simulink model "General_3_2025a"  (R2025a)
settings: Solver=ode45  StartTime=0.0  StopTime=inf  FixedStep=.1  RelTol=1e-3
undefined symbols (not defined in the file or in its folder): CR, DiscIntNeverNeededParam, LF
libraries: instrumentseriallib x3, simulink x2
settings Model: PacingRate=1000  Creator=aceve  LastModifiedBy=diego

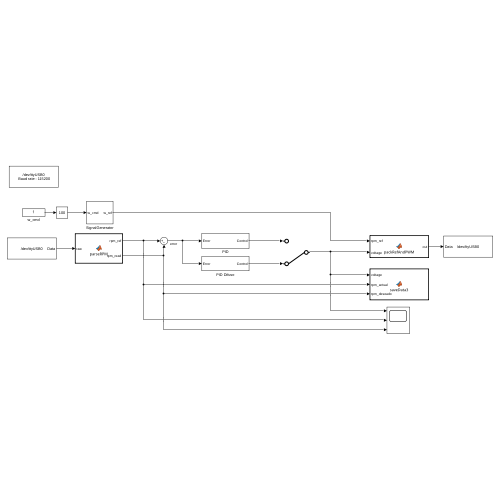
[thumbnail: Simulink's stored preview of the top-level diagram]
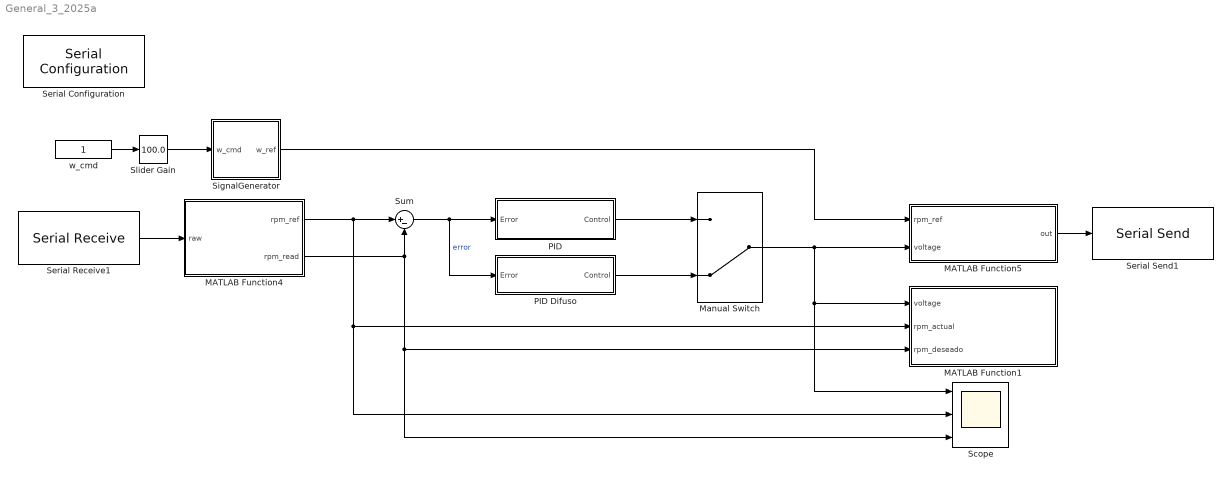
== system General_3_2025a ==
  MATLAB Function1 : MATLAB Function  TreatAsAtomicUnit=on
  MATLAB Function4 : MATLAB Function  TreatAsAtomicUnit=on
  MATLAB Function5 : MATLAB Function  TreatAsAtomicUnit=on
  Manual Switch : ManualSwitch  CurrentSetting=0
  PID : Subsystem
  PID Difuso : Subsystem
  Scope : Scope  NumInputPorts=3
      settings: ActiveDisplayYMinimum=-1  ActiveDisplayYMaximum=1
  Serial Configuration : instrumentseriallib/Serial Configuration  Priority=-200000  PortSel=/dev/ttyUSB0  Port=/dev/ttyUSB0  ComPort=/dev/ttyUSB0  BaudRate=115200  DataBits=8  Parity=none  StopBits=1  ByteOrder=little-endian  FlowControl=none  Timeout=10  SimulateUsing=Interpreted execution  BlockInModel=on  aMode=1
  Serial Receive1 : instrumentseriallib/Serial Receive  Priority=1  PortSel=/dev/ttyUSB0  Port=/dev/ttyUSB0  ComPort=/dev/ttyUSB0  DataType=int16  SaveDataType=uint8  ToggleHeader=off  Header=[]  ToggleDataSize=on  DataSize=[2 1]  ToggleTerminator=off  Terminator=CR/LF ('\r\n')  CustomTerminator=[]  InputFormat=Column major  EnableBlockingMode=on  ActionDataUnavailable=Output last received value  ActionWhenDataUnavailable=Output last received value  CustomValue=0  SampleTime=0.01  SimulateUsing=Interpreted execution  BlockInModel=on  aMode=1  LibraryInUse=instrumentlib
  Serial Send1 : instrumentseriallib/Serial Send  Priority=1  PortSel=/dev/ttyUSB0  Port=/dev/ttyUSB0  ComPort=/dev/ttyUSB0  Header=[]  Terminator=<none>  CustomTerminator=[]  EnableBlockingMode=off  SimulateUsing=Interpreted execution  BlockInModel=on  aMode=1
  SignalGenerator : Subsystem
  Slider Gain : simulink/Math Operations/Slider Gain  gain=100.0  low=100  high=1100
  Sum : Sum  Inputs=|+-
  w_cmd : Constant  SampleTime=-1
  wires:
  PID/1(Control) -> Manual Switch/1
  Sum/1 -> PID Difuso/1(Error), PID/1(Error)  "error"
  w_cmd/1 -> Slider Gain/1
  PID Difuso/1(Control) -> Manual Switch/2
  Serial Receive1/1 -> MATLAB Function4/1(raw)
  MATLAB Function5/1(out) -> Serial Send1/1
  MATLAB Function4/1(rpm_ref) -> Scope/2, MATLAB Function1/2(rpm_actual), Sum/1
  MATLAB Function4/2(rpm_read) -> Sum/2, Scope/3, MATLAB Function1/3(rpm_deseado)
  Manual Switch/1 -> Scope/1, MATLAB Function1/1(voltage), MATLAB Function5/2(voltage)
  Slider Gain/1 -> SignalGenerator/1(w_cmd)
  SignalGenerator/1(w_ref) -> MATLAB Function5/1(rpm_ref)

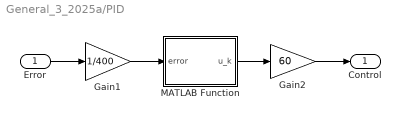
== system General_3_2025a/PID ==
  Error : Inport
  Gain1 : Gain  Gain=1/400
  Gain2 : Gain  Gain=60
  MATLAB Function : MATLAB Function  TreatAsAtomicUnit=on
  Control : Outport
  wires:
  Gain1/1 -> MATLAB Function/1(error)
  MATLAB Function/1(u_k) -> Gain2/1
  Error/1 -> Gain1/1
  Gain2/1 -> Control/1

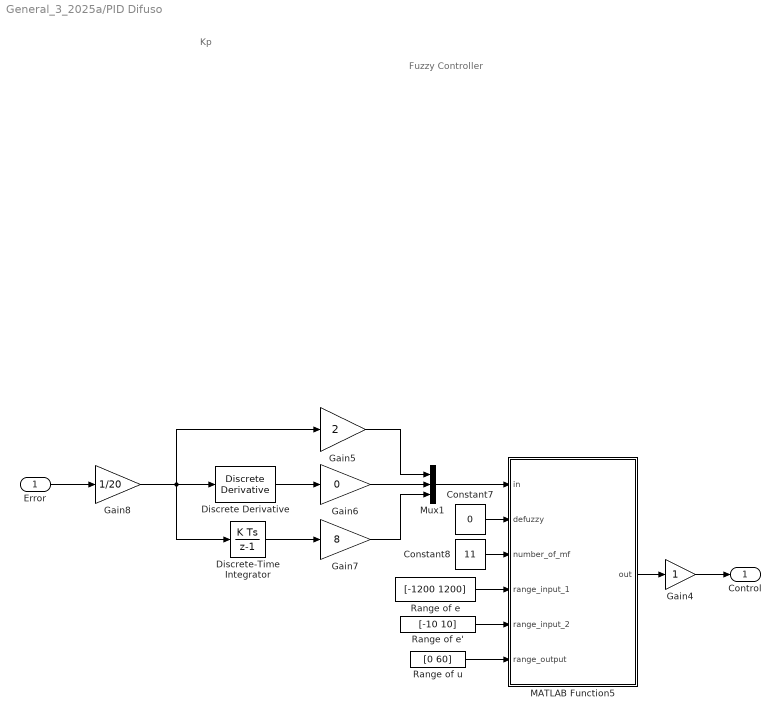
== system General_3_2025a/PID Difuso ==
  note: Fuzzy Controller
  note: Kp
  Error : Inport
  Constant7 : Constant  Value=0
  Constant8 : Constant  Value=11
  Discrete Derivative : simulink/Discrete/Discrete Derivative  gainval=1.0  ICPrevScaledInput=0.0  OutMin=[]  OutMax=[]  OutDataType=fixdt(1, 16)  OutScaling=2^-10  DoSatur=off
  Discrete-Time Integrator : DiscreteIntegrator  SampleTime=0.01  ICPrevOutput=DiscIntNeverNeededParam  ICPrevScaledInput=DiscIntNeverNeededParam
  Gain4 : Gain
  Gain5 : Gain  Gain=2
  Gain6 : Gain  Gain=0
  Gain7 : Gain  Gain=8
  Gain8 : Gain  Gain=1/20
  MATLAB Function5 : MATLAB Function  TreatAsAtomicUnit=on
  Mux1 : Mux  Inputs=3
  Range of e : Constant  Value=[-1200 1200]
  Range of e' : Constant  Value=[-10 10]
  Range of u : Constant  Value=[0 60]
  Control : Outport
  wires:
  Gain7/1 -> Mux1/3
  Range of e/1 -> MATLAB Function5/4(range_input_1)
  Gain8/1 -> Gain5/1, Discrete-Time Integrator/1, Discrete Derivative/1
  Gain6/1 -> Mux1/2
  MATLAB Function5/1(out) -> Gain4/1
  Constant8/1 -> MATLAB Function5/3(number_of_mf)
  Mux1/1 -> MATLAB Function5/1(in)
  Discrete Derivative/1 -> Gain6/1
  Discrete-Time Integrator/1 -> Gain7/1
  Range of e'/1 -> MATLAB Function5/5(range_input_2)
  Range of u/1 -> MATLAB Function5/6(range_output)
  Constant7/1 -> MATLAB Function5/2(defuzzy)
  Gain5/1 -> Mux1/1
  Gain4/1 -> Control/1
  Error/1 -> Gain8/1

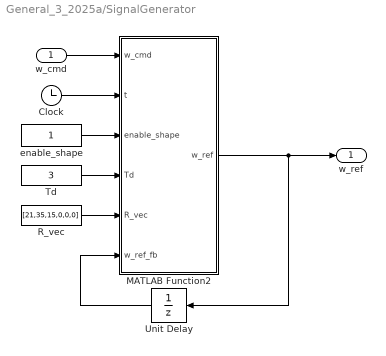
== system General_3_2025a/SignalGenerator ==
  w_cmd : Inport
  Clock : Clock
  MATLAB Function2 : MATLAB Function  TreatAsAtomicUnit=on
  R_vec : Constant  Value=[21,35,15,0,0,0]  SampleTime=-1
  Td : Constant  Value=3  SampleTime=-1
  Unit Delay : UnitDelay  SampleTime=-1  HasFrameUpgradeWarning=on
  enable_shape : Constant  SampleTime=-1
  w_ref : Outport
  wires:
  Clock/1 -> MATLAB Function2/2(t)
  Td/1 -> MATLAB Function2/4(Td)
  enable_shape/1 -> MATLAB Function2/3(enable_shape)
  Unit Delay/1 -> MATLAB Function2/6(w_ref_fb)
  R_vec/1 -> MATLAB Function2/5(R_vec)
  MATLAB Function2/1(w_ref) -> Unit Delay/1, w_ref/1
  w_cmd/1 -> MATLAB Function2/1(w_cmd)

== matlab function General_3_2025a/SignalGenerator/MATLAB Function2 ==
  settings: updateMethod=DISCRETE
  data: w_cmd input; t input; w_ref output; enable_shape input; Td input; R_vec input; w_ref_fb input
function w_ref = BezierRef(w_cmd, t, enable_shape, Td, R_vec, w_ref_fb)
% =================================================================
% VERSIÓN 5 (Coeficientes R_vec y bug de comparación corregidos)
% =================================================================
%
% Entradas:
%   w_cmd     : setpoint deseado (de la GUI)
%   t         : tiempo absoluto (Clock)
%   enable_shape : 1 = perfilar, 0 = paso directo
%   Td        : duración de la transición [s]
%   R_vec     : [r1..r6] coeficientes del polinomio
%   w_ref_fb  : w_ref anterior (feedback vía Memory/Unit Delay)
%
% Salida:
%   w_ref     : referencia suavizada

% --- estados persistentes ---
persistent w0 wf t0 last_cmd is_initialized

% --- Lógica de inicialización en el primer paso de ejecución ---
if isempty(is_initialized) || t == 0 % Se reinicia si el tiempo es 0
    is_initialized = true; 
    
    w0 = w_ref_fb; 
    wf = w_cmd;
    t0 = t;
    last_cmd = w_cmd;
end

% --- FIX 1: Detecta cambio de comando con tolerancia ---
if abs(w_cmd - last_cmd) > 1e-6
    % Nuevo tramo desde el valor de salida actual (feedback) hacia w_cmd
    w0 = w_ref_fb;
    wf = w_cmd;
    t0 = t;
    last_cmd = w_cmd;
end

% Paso directo si está desactivado
if enable_shape == 0 || Td <= 0
    w_ref = w_cmd;
    % Asegurarse de que el estado interno se actualice para el próximo arranque
    w0 = w_cmd; 
    wf = w_cmd;
    last_cmd = w_cmd;
    return
end

% Progreso normalizado en [0,1]
s = (t - t0) / Td;

if s <= 0
    alpha = 0;
elseif s >= 1
    alpha = 1;
else
    % Bezier polinómico
    if numel(R_vec) < 6
        alpha = s; % Fallback a rampa lineal
    else
        % --- FIX 2: Validar que R_vec sea correcto ---
        % La suma de coeficientes alternados debe ser 1 para que alpha(1)=1.
        % (r1 - r2 + r3 - r4 + r5 - r6) == 1
        % Si no, se usa una rampa simple s^5.
        
        r1 = R_vec(1); r2 = R_vec(2); r3 = R_vec(3);
        r4 = R_vec(4); r5 = R_vec(5); r6 = R_vec(6);
        
        % Comprobamos si el vector R_vec está mal (la suma es != 1)
        if abs((r1 - r2 + r3 - r4 + r5 - r6) - 1.0) > 1e-3
            % Vector R_vec incorrecto. Usar rampa s^5 simple.
            alpha = s^5;
        else
            % Vector R_vec es válido, usar la fórmula completa
            alpha = (s.^5).*(r1 - r2*s + r3*s.^2 - r4*s.^3 + r5*s.^4 - r6*s.^5);
        end
    end
    
    % Clampeo por seguridad numérica
    if alpha < 0, alpha = 0; end
    if alpha > 1, alpha = 1; end
end

% Interpolación entre w0 y wf
w_ref = w0 + alpha*(wf - w0);

== matlab function General_3_2025a/MATLAB Function4 ==
  data: rpm_ref output; raw input; rpm_read output
function [rpm_ref, rpm_read] = parseRPM(raw)
%#codegen
% raw: 1x2 uint16 vector received from ESP32
% rpm_read: measured RPM from encoder
% rpm_ref:  reference RPM echoed back from ESP32

rpm_read = double(raw(1));   % first  uint16 from ESP32
rpm_ref  = double(raw(2));   % second uint16 from ESP32
end

== matlab function General_3_2025a/MATLAB Function1 ==
  data: voltage input; rpm_actual input; rpm_deseado input
function saveData3(voltage, rpm_actual, rpm_deseado)
assignin('base','rpm_actual',  rpm_actual);
assignin('base','rpm_deseado', rpm_deseado);
assignin('base','voltage',     voltage);
end

== matlab function General_3_2025a/PID Difuso/MATLAB Function5 ==
  data: in input; out output; defuzzy input; number_of_mf input; range_input_1 input; range_input_2 input; range_output input
function out = fcn(in, defuzzy, number_of_mf, range_input_1, range_input_2, range_output)
% CONTROLADOR FUZZY PID (Fuzzy PD + I)
% in: [error_scaled, d_error_scaled, integral_scaled]
% defuzzy: 0 = COG, 1 = CA
% range_input_1/2: [min, max] (Universo para PD)
% range_output: [min, max] (Universo para Salida Final, ej: [6, 54])

% === 1. Preparar divisiones ===
n = number_of_mf;
div1 = linspace(range_input_1(1), range_input_1(2), n); % error
div2 = linspace(range_input_2(1), range_input_2(2), n); % d_error

% El universo de salida del PD difuso. 
% Lo definimos igual que el rango de salida final por simplicidad.
div_out = linspace(range_output(1), range_output(2), n);

% === 2. Calcular membresías de entrada (solo para PD) ===
mu_e = compute_memberships(in(1), div1);
mu_de = compute_memberships(in(2), div2);

% === 3. Definir FAM (PD) ===
FAM = zeros(n, n);
middle_val = (n + 1) / 2;
middle_ij = middle_val*2;
for i = 1:n
    for j = 1:n
        v = middle_val + middle_ij - (i + j);
        if v > n, v = n; end
        if v < 1, v = 1; end
        FAM(i,j) = v;
    end
end

% === 4. Activaciones de reglas (PD) ===
rule_heights = zeros(n,n);
for i = 1:n
    for j = 1:n
        h = min(mu_e(i), mu_de(j));
        rule_heights(i,j) = h;
    end
end
% Max activación por salida
mu_out = zeros(1,n);
for k = 1:n
    % Encuentra todas las reglas (i,j) que tienen la salida k
    mask = (FAM == k);
    if any(mask(:)) % Evita max([]) si una etiqueta de salida no se usa
        mu_out(k) = max(rule_heights(mask));
    else
        mu_out(k) = 0;
    end
end

% === 5. Defuzzificación (Cálculo de la Salida PD) ===
% Usamos un valor central robusto por si den == 0
midL = floor((n+1)/2);
midR = ceil((n+1)/2);
center_val = 0.5*(div_out(midL) + div_out(midR));

fuzzy_pd_out = center_val; % Valor por defecto

if defuzzy == 0
    % --- COG (Centroide) ---
    num = 0; den = 0;
    if n > 1
        step = div_out(2)-div_out(1);
    else
        step = 0; % Evitar error si n=1
    end
    base = 2*step; % base total de cada triángulo
    for k = 1:n
        h = mu_out(k);
        if h > 0
            top_base = (1-h)*base;
            A = h*(base+top_base)/2; % área del trapecio
            num = num + A*div_out(k);
            den = den + A;
        end
    end
    if den > eps
        fuzzy_pd_out = num/den;
    end
else
    % --- CA (Promedio Ponderado) ---
    num = sum(mu_out .* div_out);
    den = sum(mu_out);
    if den > eps
        fuzzy_pd_out = num/den;
    end
end

% === 6. COMBINACIÓN PID (Fuzzy PD + I) ===
% Sumamos la salida difusa PD con la entrada Integral (in(3))
out_unclamped = fuzzy_pd_out + in(3);

% === 7. SATURACIÓN DE SALIDA ===
% Forzamos la salida final a estar dentro del rango [6, 54]
if out_unclamped < range_output(1)
    out = range_output(1); % Mínimo 6V
elseif out_unclamped > range_output(2)
    out = range_output(2); % Máximo 54V
else
    out = out_unclamped;
end

end

% === Función Auxiliar de Membresías ===
function mu = compute_memberships(x, div)
n = length(div);
mu = zeros(1,n);
if x <= div(1)
    mu(1) = 1; return
elseif x >= div(end)
    mu(end) = 1; return
end
for i = 1:n-1
    x1 = div(i); x2 = div(i+1);
    den = x2 - x1;
    if den == 0, den = eps; end % Evitar división por cero
    
    if x >= x1 && x <= x2
        mu(i) = (x2 - x)/den;
        mu(i+1) = (x - x1)/den;
        return
    end
end
end

== matlab function General_3_2025a/MATLAB Function5 ==
  data: rpm_ref input; voltage input; out output
function out = packRefAndPWM(rpm_ref, voltage)
v_min = 0;
v_max = 60;

pwm_min = 0;
pwm_max = 65535;

% Escalado lineal
pwm_raw = (voltage - v_min) * (pwm_max - pwm_min) / (v_max - v_min) + pwm_min;

% Saturación
if pwm_raw > pwm_max * 0.9
    pwm_raw = pwm_max * 0.9;
elseif pwm_raw < pwm_max * 0.1
    pwm_raw = pwm_max * 0.1;
end

pwm_u16 = uint16(pwm_raw);
rpm_ref_u16 = uint16(rpm_ref);

out = uint16([rpm_ref_u16, pwm_u16]);
end

== matlab function General_3_2025a/PID/MATLAB Function ==
  data: error input; u_k output
function u_k = PID(error)
% Esta función implementa el controlador PID discreto del código de Arduino.
% ENTRADA:
%   error: El error actual e(k) = (referencia - medida)
% SALIDA:
%   u_k: La señal de control saturada (entre 0.0 y 1.0)

% ===== Parámetros del Controlador (iguales a los de Arduino) =====
Kc = 0.12;
Ti = 0.05;
Td = 0.005;
N = 100;
Ts_s = 0.01; % Periodo de muestreo en segundos (20 ms)

% ===== Variables de Estado (persisten entre llamadas) =====
% Se declaran como 'persistent' para que guarden su valor,
% igual que las variables globales en Arduino.
persistent error_prev integral_prev derivative_prev

% ===== Inicialización en la primera ejecución =====
% La primera vez que se llama a la función, las variables están vacías.
if isempty(error_prev)
    error_prev = 0.0;
    integral_prev = 0.0;
    derivative_prev = 0.0;
end

% ================================================================
% ===== LÓGICA DE CONTROL PID (Traducción directa de C++) ========
% ================================================================

% 2. Calcular término Proporcional: p(k) = Kc * e(k)
p_k = Kc * error;

% 3. Calcular término Integral: i(k) = i(k-1) + (h*Kc/Ti) * e(k)
i_k = integral_prev + (Kc * Ts_s / Ti) * error;

% 4. Calcular término Derivativo: d(k) = c1*d(k-1) + c2*e(k) - c2*e(k-1)
c1 = 1.0 / (1.0 + Ts_s * N);
c2 = (Kc * Td * N) / (1.0 + Ts_s * N);
d_k = c1 * derivative_prev + c2 * (error - error_prev);

% 5. Calcular la salida de control total: u(k) = p(k) + i(k) + d(k)
u_k_total = p_k + i_k + d_k;

% --- Saturación y Anti-Windup ---
u_k_saturado = u_k_total;
if u_k_saturado > 1.0
    u_k_saturado = 1.0;
end
if u_k_saturado < 0.0
    u_k_saturado = 0.0;
end

% --- Actualización de estados para la siguiente iteración ---
% Anti-Windup: Actualizar el término integral solo si no hay saturación
if u_k_total == u_k_saturado
    integral_prev = i_k;
end
derivative_prev = d_k;
error_prev = error;

% Asignar la salida final de la función
u_k = u_k_saturado;

end
